simulink model "follow"  (R2021b)
settings: Solver=VariableStepAuto  StartTime=0.0  StopTime=100  RelTol=1e-3
libraries: simulink x1
settings Model: Creator=84232  LastModifiedBy=84232

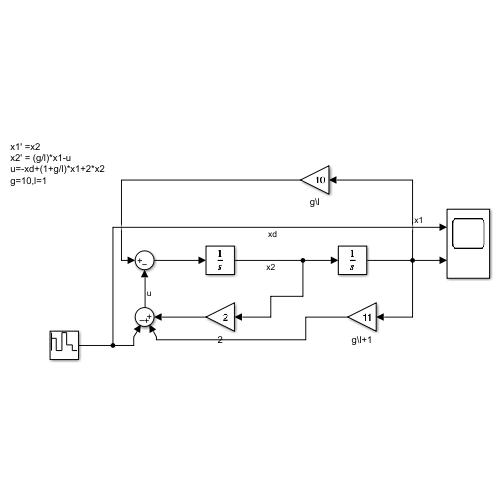
[thumbnail: Simulink's stored preview of the top-level diagram]
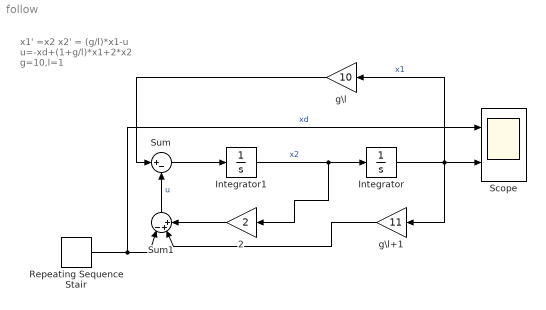
== system follow ==
  note: x1' =x2
      | x2' = (g/l)*x1-u
      | u=-xd+(1+g/l)*x1+2*x2
      | g=10,l=1
  2 : Gain  Gain=2
  Integrator : Integrator
  Integrator1 : Integrator
  Repeating Sequence Stair : simulink/Sources/Repeating Sequence Stair  OutValues=[3 1 4 2 1].'  tsamp=20  OutMin=[]  OutMax=[]  OutDataTypeStr=double  OutputDataTypeScalingMode=double  OutDataType=fixdt(0,8)  ConRadixGroup=Best Precision: Vector-wise  OutScaling=2^-12
  Scope : Scope  NumInputPorts=2
  Sum : Sum  Inputs=|+-
  Sum1 : Sum  Inputs=|-++
  g\l : Gain  Gain=10
  g\l+1 : Gain  Gain=11
  wires:
  Integrator1/1 -> 2/1, Integrator/1  "x2"
  Integrator/1 -> g\l/1, Scope/2, g\l+1/1  "x1"
  g\l/1 -> Sum/1
  Sum/1 -> Integrator1/1
  Sum1/1 -> Sum/2  "u"
  g\l+1/1 -> Sum1/2
  2/1 -> Sum1/3
  Repeating Sequence Stair/1 -> Scope/1, Sum1/1  "xd"
